simulink subsystem "LQR_classical"  (R2024a)
settings: Solver=VariableStepAuto  StartTime=0.0  StopTime=10.0  RelTol=1e-3
undefined symbols (not defined in the file): K_LQR_classical, u_eq, x_eq
settings Model: Creator=Bocchio  LastModifiedBy=Bocchio

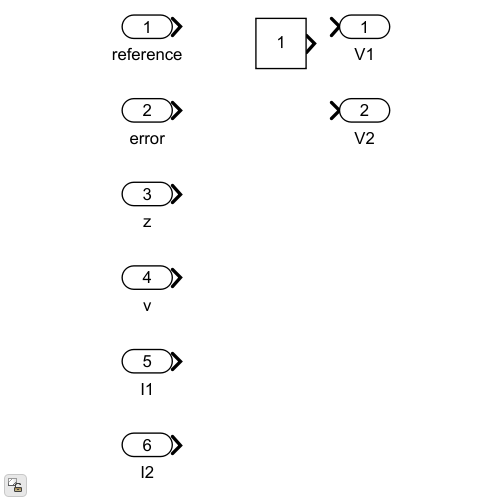
[thumbnail: Simulink's stored preview of the top-level diagram]
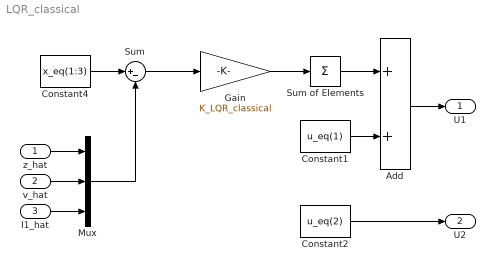
== system LQR_classical ==
  z_hat : Inport
  v_hat : Inport  Port=2
  I1_hat : Inport  Port=3
  Add : Sum
  Constant1 : Constant  Value=u_eq(1)
  Constant2 : Constant  Value=u_eq(2)
  Constant4 : Constant  Value=x_eq(1:3)
  Gain : Gain  Gain=K_LQR_classical
  Mux : Mux  Inputs=3
  Sum : Sum  Inputs=|+-
  Sum of Elements : Sum  Inputs=+  CollapseDim=2
  U1 : Outport
  U2 : Outport  Port=2
  wires:
  Gain/1 -> Sum of Elements/1
  Constant1/1 -> Add/2
  z_hat/1 -> Mux/1
  v_hat/1 -> Mux/2
  I1_hat/1 -> Mux/3
  Constant4/1 -> Sum/1
  Mux/1 -> Sum/2
  Sum/1 -> Gain/1
  Sum of Elements/1 -> Add/1
  Add/1 -> U1/1
  Constant2/1 -> U2/1
